simulink model "dh_thuan_cg_0521"  (R2018a)
settings: Solver=VariableStepAuto  StartTime=0.0  StopTime=10.0  RelTol=1e-3
settings Model: Creator=Nguyen Mai  LastModifiedBy=Nguyen Mai

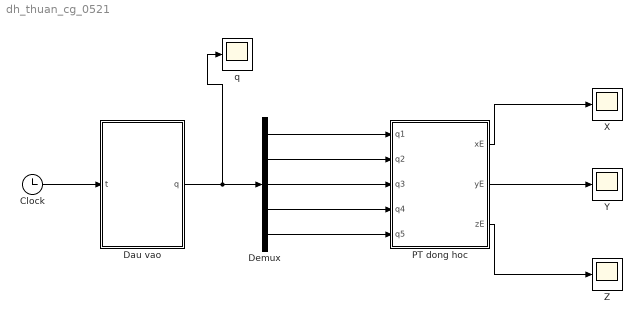
== system dh_thuan_cg_0521 ==
  Clock : Clock
  Dau vao : MATLAB Function  TreatAsAtomicUnit=on
  Demux : Demux  Outputs=5
  PT dong hoc : MATLAB Function  TreatAsAtomicUnit=on
  X : Scope
  Y : Scope
  Z : Scope
  q : Scope
  wires:
  PT dong hoc/2(yE) -> Y/1
  PT dong hoc/1(xE) -> X/1
  PT dong hoc/3(zE) -> Z/1
  Clock/1 -> Dau vao/1(t)
  Dau vao/1(q) -> q/1, Demux/1
  Demux/1 -> PT dong hoc/1(q1)
  Demux/2 -> PT dong hoc/2(q2)
  Demux/3 -> PT dong hoc/3(q3)
  Demux/4 -> PT dong hoc/4(q4)
  Demux/5 -> PT dong hoc/5(q5)

== matlab function dh_thuan_cg_0521/PT dong hoc ==
  data: q1 input; xE output; yE output; zE output; q2 input; q3 input; q4 input; q5 input
function [xE,yE, zE] = fcn(q1,q2,q3,q4,q5)
L2 = 0.5;
L3 = 0.2;
L4 = 0.2;
L5 = 0.5;
xE=-L5 * cos(q4) * cos(q1) * sin(q3) * cos(q5) + L5 * sin(q4) * sin(q1) * cos(q5) - cos(q1) * cos(q3) * L5 * sin(q5) + cos(q1) * L3 * cos(q3) + cos(q1) * cos(q3) * L4 + cos(q1) * L2;
yE=-L5 * cos(q4) * sin(q1) * sin(q3) * cos(q5) - L5 * sin(q4) * cos(q1) * cos(q5) - sin(q1) * cos(q3) * L5 * sin(q5) + sin(q1) * L3 * cos(q3) + sin(q1) * cos(q3) * L4 + sin(q1) * L2;
zE=cos(q3) * cos(q4) * L5 * cos(q5) - sin(q3) * L5 * sin(q5) + sin(q3) * L4 + L3 * sin(q3) + q2;
end

== matlab function dh_thuan_cg_0521/Dau vao ==
  data: t input; q output
function q  = fcn(t)
q1=sin(t);
q2=0.07*t;
q3=cos(t);
q4=0.25*sin(t);
q5=0.75*cos(t);
q=zeros(5,1);
q(1,1)=q1;
q(2,1)=q2;
q(3,1)=q3;
q(4,1)=q4;
q(5,1)=q5;
end
